simulink model "f16controls"  (R2024b)
settings: Solver=VariableStepAuto  StartTime=0.0  StopTime=1  RelTol=1e-3
settings Model: Creator=MSI  LastModifiedBy=MSI

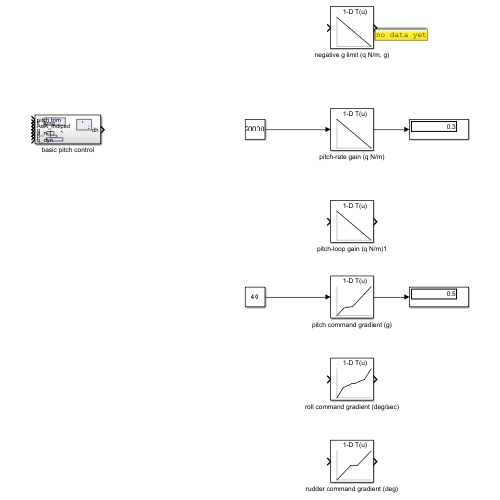
[thumbnail: Simulink's stored preview of the top-level diagram]
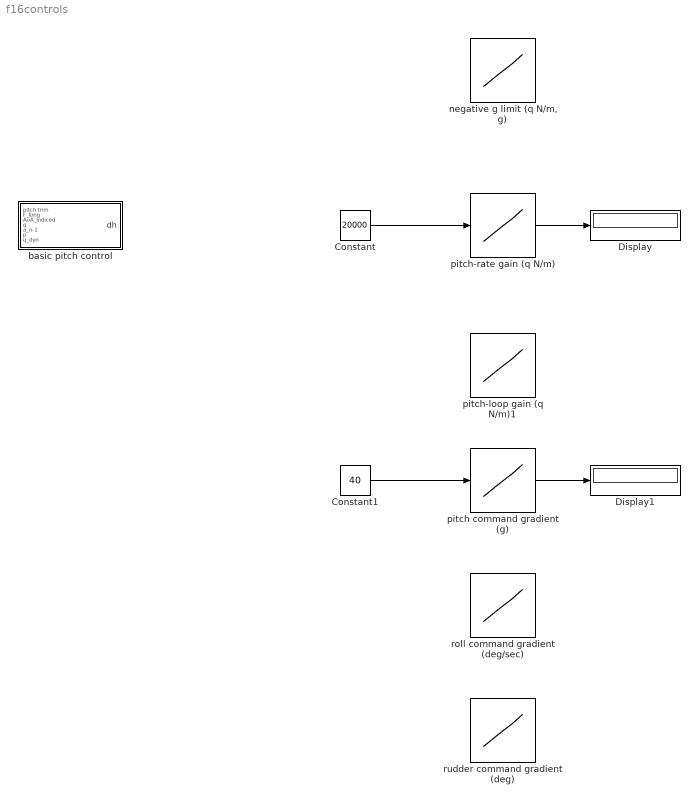
== system f16controls ==
  Constant : Constant  Value=20000
  Constant1 : Constant  Value=40
  Display : Display
  Display1 : Display
  basic pitch control : Subsystem
  "negative g limit (q N/m, g)" : Lookup_n-D  NumberOfTableDimensions=1  BreakpointsForDimension1=[2000, 9000]  Table=[-1, -4]  ExtrapMethod=Clip  UseLastTableValue=on  InternalRulePriority=Speed  RndMeth=Simplest
  pitch command gradient (g) : Lookup_n-D  NumberOfTableDimensions=1  BreakpointsForDimension1=[-80, -30, -10, 10, 40, 180]  Table=[-4, -0.6, 0, 0, 0.5, 10]  ExtrapMethod=Clip  UseLastTableValue=on  InternalRulePriority=Speed  RndMeth=Simplest
  pitch-loop gain (q N/m)1 : Lookup_n-D  NumberOfTableDimensions=1  BreakpointsForDimension1=[14000, 42000]  Table=[1, 0.4]  ExtrapMethod=Clip  UseLastTableValue=on  InternalRulePriority=Speed  RndMeth=Simplest
  pitch-rate gain (q N/m) : Lookup_n-D  NumberOfTableDimensions=1  BreakpointsForDimension1=[6000, 15000]  Table=[1, 0.3]  ExtrapMethod=Clip  UseLastTableValue=on  InternalRulePriority=Speed  RndMeth=Simplest
  roll command gradient (deg/sec) : Lookup_n-D  NumberOfTableDimensions=1  BreakpointsForDimension1=[-80, -50, -25, -8, 8, 25, 50, 80]  Table=[-330, -90, -40, 0, 0, 40, 90, 330]  ExtrapMethod=Clip  UseLastTableValue=on  InternalRulePriority=Speed  RndMeth=Simplest
  rudder command gradient (deg) : Lookup_n-D  NumberOfTableDimensions=1  BreakpointsForDimension1=[-500, -90, 90, 500]  Table=[-30, 0, 0, 30]  ExtrapMethod=Clip  UseLastTableValue=on  InternalRulePriority=Speed  RndMeth=Simplest
  wires:
  Constant/1 -> pitch-rate gain (q N/m)/1
  pitch-rate gain (q N/m)/1 -> Display/1
  Constant1/1 -> pitch command gradient (g)/1
  pitch command gradient (g)/1 -> Display1/1

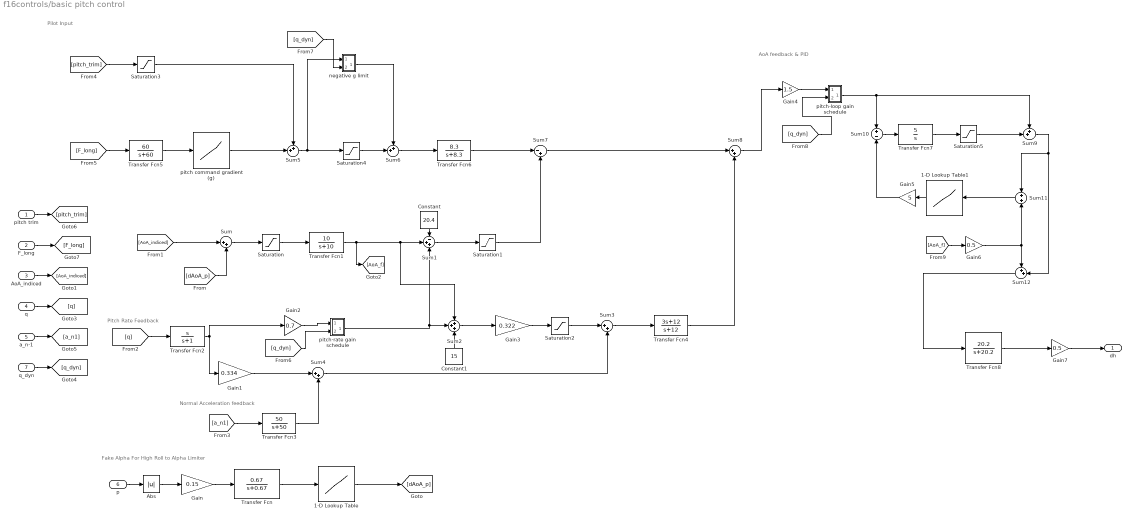
== system f16controls/basic pitch control ==
  note: AoA feedback & PID
  note: Pilot Input
  note: Normal Acceleration feedback
  note: Pitch Rate Feedback
  note: Fake Alpha For High Roll to Alpha Limiter
  pitch trim : Inport
  F_long : Inport  Port=2
  AoA_indiced : Inport  Port=3
  q : Inport  Port=4
  a_n-1 : Inport  Port=5
  p : Inport  Port=6
  q_dyn : Inport  Port=7
  1-D Lookup Table : Lookup_n-D  NumberOfTableDimensions=1  BreakpointsForDimension1=[3, 8.4]  Table=[0, 5.4]  ExtrapMethod=Clip  UseLastTableValue=on  InternalRulePriority=Speed  RndMeth=Simplest
  1-D Lookup Table1 : Lookup_n-D  NumberOfTableDimensions=1  BreakpointsForDimension1=[-25, 25]  Table=[0, 0]  InternalRulePriority=Speed  RndMeth=Simplest
  Abs : Abs  SaturateOnIntegerOverflow=off
  Constant : Constant  Value=20.4
  Constant1 : Constant  Value=15
  Gain : Gain  Gain=0.15
  Gain1 : Gain  Gain=0.334
  Gain2 : Gain  Gain=0.7
  Gain3 : Gain  Gain=0.322
  Gain4 : Gain  Gain=1.5
  Gain5 : Gain  Gain=5
  Gain6 : Gain  Gain=0.5
  Gain7 : Gain  Gain=0.5
  Saturation : Saturate  UpperLimit=30  LowerLimit=-5
  Saturation1 : Saturate  UpperLimit=inf  LowerLimit=0
  Saturation2 : Saturate  UpperLimit=inf  LowerLimit=0
  Saturation3 : Saturate  UpperLimit=2.4  LowerLimit=-2.4
  Saturation4 : Saturate  UpperLimit=8  LowerLimit=0
  Saturation5 : Saturate  UpperLimit=25  LowerLimit=-25
  Sum{,3..4,8} (4 alike) : Sum  Inputs=|++
  Sum1 : Sum  Inputs=-++
  Sum10 : Sum  Inputs=+-
  Sum11 : Sum
  Sum{5..6,9,12} (4 alike) : Sum  Inputs=++|
  Sum2 : Sum  Inputs=+++
  Sum7 : Sum  Inputs=|-+
  Transfer Fcn : TransferFcn  Numerator=[0.67]  Denominator=[1 0.67]
  Transfer Fcn1 : TransferFcn  Numerator=[10]  Denominator=[1 10]
  Transfer Fcn2 : TransferFcn  Numerator=[1 0]  Denominator=[1 1]
  Transfer Fcn3 : TransferFcn  Numerator=[50]  Denominator=[1 50]
  Transfer Fcn4 : TransferFcn  Numerator=[3 12]  Denominator=[1 12]
  Transfer Fcn5 : TransferFcn  Numerator=[60]  Denominator=[1 60]
  Transfer Fcn6 : TransferFcn  Numerator=[8.3]  Denominator=[1 8.3]
  Transfer Fcn7 : TransferFcn  Numerator=[5]  Denominator=[1 0]
  Transfer Fcn8 : TransferFcn  Numerator=[20.2]  Denominator=[1 20.2]
  negative g limit : Subsystem
  pitch command gradient (g) : Lookup_n-D  NumberOfTableDimensions=1  BreakpointsForDimension1=[-80, -30, -10, 10, 40, 180]  Table=[-4, -0.6, 0, 0, 0.5, 10]  ExtrapMethod=Clip  UseLastTableValue=on  InternalRulePriority=Speed  RndMeth=Simplest
  pitch-loop gain schedule : Subsystem
  pitch-rate gain schedule : Subsystem
  dh : Outport
  wires:
  p/1 -> Abs/1
  Abs/1 -> Gain/1
  Gain/1 -> Transfer Fcn/1
  Transfer Fcn/1 -> 1-D Lookup Table/1
  1-D Lookup Table/1 -> [dAoA_p]
  AoA_indiced/1 -> [AoA_indiced]
  [AoA_indiced] -> Sum/1
  [dAoA_p] -> Sum/2
  Sum/1 -> Saturation/1
  Saturation/1 -> Transfer Fcn1/1
  q/1 -> [q]
  [q] -> Transfer Fcn2/1
  Transfer Fcn2/1 -> Gain2/1, Gain1/1
  Gain1/1 -> Sum4/1
  q_dyn/1 -> [q_dyn]
  Gain2/1 -> pitch-rate gain schedule/1(In1)
  pitch-rate gain schedule/1(Out1) -> Sum2/2, Sum1/3
  Constant/1 -> Sum1/1
  Sum1/1 -> Saturation1/1
  Saturation1/1 -> Sum7/2
  Transfer Fcn1/1 -> [AoA_f], Sum2/1, Sum1/2
  Constant1/1 -> Sum2/3
  Sum2/1 -> Gain3/1
  Gain3/1 -> Saturation2/1
  Saturation2/1 -> Sum3/1
  a_n-1/1 -> [a_n1]
  [a_n1] -> Transfer Fcn3/1
  Transfer Fcn3/1 -> Sum4/2
  Sum4/1 -> Sum3/2
  Sum3/1 -> Transfer Fcn4/1
  Transfer Fcn4/1 -> Sum8/2
  pitch trim/1 -> [pitch_trim]
  [pitch_trim] -> Saturation3/1
  Saturation3/1 -> Sum5/1
  F_long/1 -> [F_long]
  [F_long] -> Transfer Fcn5/1
  Transfer Fcn5/1 -> pitch command gradient (g)/1
  pitch command gradient (g)/1 -> Sum5/2
  Sum5/1 -> negative g limit/1(In1), Saturation4/1
  Saturation4/1 -> Sum6/2
  negative g limit/1(Out1) -> Sum6/1
  [q_dyn] -> pitch-rate gain schedule/2(Input)
  [q_dyn] -> negative g limit/2(Input)
  Sum6/1 -> Transfer Fcn6/1
  Transfer Fcn6/1 -> Sum7/1
  Sum7/1 -> Sum8/1
  Sum8/1 -> Gain4/1
  [q_dyn] -> pitch-loop gain schedule/2(Input)
  Gain4/1 -> pitch-loop gain schedule/1(In1)
  pitch-loop gain schedule/1(Out1) -> Sum10/1, Sum9/1
  Sum10/1 -> Transfer Fcn7/1
  Transfer Fcn7/1 -> Saturation5/1
  Saturation5/1 -> Sum9/2
  Sum9/1 -> Sum11/1, Sum12/2
  Gain6/1 -> Sum11/2, Sum12/1
  Sum11/1 -> 1-D Lookup Table1/1
  Gain5/1 -> Sum10/2
  1-D Lookup Table1/1 -> Gain5/1
  [AoA_f] -> Gain6/1
  Sum12/1 -> Transfer Fcn8/1
  Transfer Fcn8/1 -> Gain7/1
  Gain7/1 -> dh/1

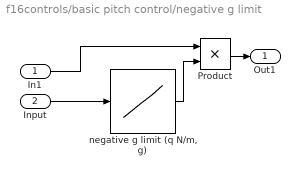
== system f16controls/basic pitch control/negative g limit ==
  In1 : Inport
  Input : Inport  Port=2
  Product : Product
  "negative g limit (q N/m, g)" : Lookup_n-D  NumberOfTableDimensions=1  BreakpointsForDimension1=[2000, 9000]  Table=[-1, -4]  ExtrapMethod=Clip  UseLastTableValue=on  InternalRulePriority=Speed  RndMeth=Simplest
  Out1 : Outport
  wires:
  Input/1 -> "negative g limit (q N/m, g)"/1
  "negative g limit (q N/m, g)"/1 -> Product/2
  Product/1 -> Out1/1
  In1/1 -> Product/1

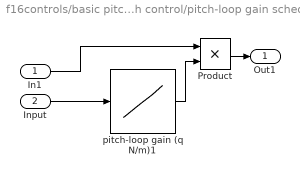
== system f16controls/basic pitch control/pitch-loop gain schedule ==
  In1 : Inport
  Input : Inport  Port=2
  Product : Product
  pitch-loop gain (q N/m)1 : Lookup_n-D  NumberOfTableDimensions=1  BreakpointsForDimension1=[14000, 42000]  Table=[1, 0.4]  ExtrapMethod=Clip  UseLastTableValue=on  InternalRulePriority=Speed  RndMeth=Simplest
  Out1 : Outport
  wires:
  Input/1 -> pitch-loop gain (q N/m)1/1
  pitch-loop gain (q N/m)1/1 -> Product/2
  Product/1 -> Out1/1
  In1/1 -> Product/1

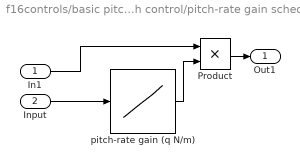
== system f16controls/basic pitch control/pitch-rate gain schedule ==
  In1 : Inport
  Input : Inport  Port=2
  Product : Product
  pitch-rate gain (q N/m) : Lookup_n-D  NumberOfTableDimensions=1  BreakpointsForDimension1=[6000, 15000]  Table=[1, 0.3]  ExtrapMethod=Clip  UseLastTableValue=on  InternalRulePriority=Speed  RndMeth=Simplest
  Out1 : Outport
  wires:
  Input/1 -> pitch-rate gain (q N/m)/1
  pitch-rate gain (q N/m)/1 -> Product/2
  Product/1 -> Out1/1
  In1/1 -> Product/1
